simulink model "Simulink Circuit Design"  (R2024b)
settings: Solver=VariableStepAuto  StartTime=0.0  StopTime=1  RelTol=1e-3
libraries: spsSeriesRLCBranchLib x28, spsMosfetLib x24, spsVoltageMeasurementLib x10, spsCurrentMeasurementLib x7, spsDCVoltageSourceLib x4, spsGroundLib x1, sps_lib x1, spspowerguiLib x1
settings Model: Creator=davut.ertekin  LastModifiedBy=jraza
settings SolverCC: ZeroCrossAlgorithm=Adaptive
settings DebuggingCC: IgnoredZcDiagnostic=none
settings RTWCC: GPUComputeCapability=3.5

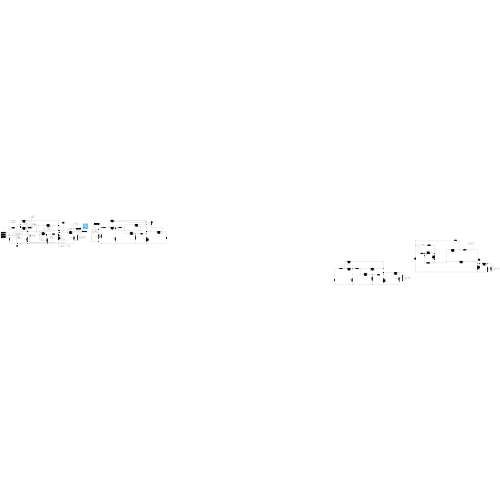
[thumbnail: Simulink's stored preview of the top-level diagram]
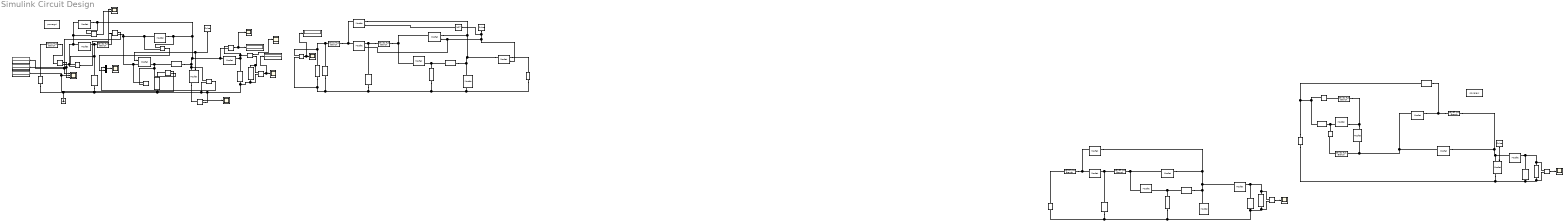
== system Simulink Circuit Design ==
  Co{3..4,8,14,16,19,21} (7 alike) : spsSeriesRLCBranchLib/Series RLC Branch  LConnTagsString=__new0  RConnTagsString=__new0  BranchType=C  Resistance=1  Inductance=1e-3  SetiL0=off  InitialCurrent=0  Capacitance=470e-6  Setx0=off  InitialVoltage=0  Measurements=None
  Co{2,5,9,15,20} (5 alike) : spsSeriesRLCBranchLib/Series RLC Branch  LConnTagsString=__new0  RConnTagsString=__new0  BranchType=C  Resistance=1  Inductance=1e-3  SetiL0=off  InitialCurrent=0  Capacitance=100e-6  Setx0=off  InitialVoltage=0  Measurements=None
  Current Measurement{,1..6} (7 alike) : spsCurrentMeasurementLib/Current Measurement  PhasorSimulation=off  OutputType=Complex  PSBequivalent=0
  DC Voltage Source : spsDCVoltageSourceLib/DC Voltage Source  Amplitude=300  Measurements=None
  DC Voltage Source2 : spsDCVoltageSourceLib/DC Voltage Source  Amplitude=24  Measurements=None
  DC Voltage Source4 : spsDCVoltageSourceLib/DC Voltage Source  Amplitude=24  Measurements=None
  DC Voltage Source6 : spsDCVoltageSourceLib/DC Voltage Source  Amplitude=24  Measurements=None
  Display{,1..5} (6 alike) : Display
  Ground : spsGroundLib/Ground  LConnTagsString=a
  L{1..3,7..9,14..15,17,19..21} (12 alike) : spsSeriesRLCBranchLib/Series RLC Branch  LConnTagsString=__new0  RConnTagsString=__new0  BranchType=L  Resistance=1  Inductance=330e-6  SetiL0=off  InitialCurrent=0  Capacitance=1e-6  Setx0=off  InitialVoltage=0  Measurements=None
  Load2 : spsSeriesRLCBranchLib/Series RLC Branch  LConnTagsString=__new0  RConnTagsString=__new0  BranchType=R  Resistance=200  Inductance=1e-3  SetiL0=off  InitialCurrent=0  Capacitance=1e-6  Setx0=off  InitialVoltage=0  Measurements=None
  Load3 : spsSeriesRLCBranchLib/Series RLC Branch  LConnTagsString=__new0  RConnTagsString=__new0  BranchType=R  Resistance=50  Inductance=1e-3  SetiL0=off  InitialCurrent=0  Capacitance=1e-6  Setx0=off  InitialVoltage=0  Measurements=None
  Load5 : spsSeriesRLCBranchLib/Series RLC Branch  LConnTagsString=__new0  RConnTagsString=__new0  BranchType=R  Resistance=300  Inductance=1e-3  SetiL0=off  InitialCurrent=0  Capacitance=1e-6  Setx0=off  InitialVoltage=0  Measurements=None
  Load7 : spsSeriesRLCBranchLib/Series RLC Branch  LConnTagsString=__new0  RConnTagsString=__new0  BranchType=R  Resistance=200  Inductance=1e-3  SetiL0=off  InitialCurrent=0  Capacitance=1e-6  Setx0=off  InitialVoltage=0  Measurements=None
  Mosfet{1..6,13..18,27..32,37..42} (24 alike) : spsMosfetLib/Mosfet  Ron=0.01  Lon=0  Rd=0.01  Vfd=0  IC=0  Rs=1e5  Cs=inf  Measurements=on
  Mux : Mux  Inputs=2
  NOT : Logic  Operator=NOT  IconShape=distinctive  AllPortsSameDT=off  OutDataTypeStr=boolean
  Pulse Generator1 : DiscretePulseGenerator  PulseType=Time based  Period=1/50000  PulseWidth=43
  Pulse Generator3 : DiscretePulseGenerator  PulseType=Time based  Period=1/50000  PulseWidth=80
  Pulse Generator4 : DiscretePulseGenerator  PulseType=Time based  Period=1/50000  PulseWidth=50.005
  Scope{,1,3..5,7..9} (8 alike) : Scope
  Scope2 : Scope  NumInputPorts=3
  Scope6 : Scope  NumInputPorts=2
  Vo{2..3,5,7} (4 alike) : spsVoltageMeasurementLib/Voltage Measurement  PhasorSimulation=off  OutputType=Complex  PSBequivalent=0
  Voltage Measurement{,1..5} (6 alike) : spsVoltageMeasurementLib/Voltage Measurement  PhasorSimulation=off  OutputType=Complex  PSBequivalent=0
  powergui : sps_lib/powergui  Priority=1  SimulationMode=Discrete  SampleTime=2e-6  frequency=60  Iterations=50  frequencyindice=0  Pbase=100e6  ErrMax=1e-4  UnitsV=kV  UnitsW=MW  buscounter=0  FunctionMessages=off  echomessages=off  EnableUseOfTLC=off  CurrentSourceSwitches=off  DisableSnubberDevices=off  DisableRonSwitches=off  DisableVfSwitches=off  DisplayEquations=off  AutomaticDiscreteSolvers=off  SolverType=Tustin/Backward Euler (TBE)  Interpol=off  ExternalGateDelay=off  methode=off  Ts=100  x0status=blocks  SPID=on  SwTol=0  HookPort=off  NonlinearTolerance=1e-4  nMaxIteration=100  ContinueOnMaxIteration=off  RestoreLinks=warning  ResistiveCurrentMeasurement=off  Frange=[0:2:500]  Ylog=off  Xlog=on  ShowGrid=off  save=off  variable=ZData  structure=0  ZoomFFT=off  StartTime=0.0  cycles=1  DisplayStyle=1  fundamental=60  FreqAxis=off  MaxFrequency=1000  frequencyindicesteady=1  RmsSteady=1  display=off
  powergui2 : spspowerguiLib/powergui  Priority=1  SimulationMode=Continuous  SampleTime=50e-6  frequency=60  Iterations=50  frequencyindice=0  Pbase=100e6  ErrMax=1e-4  UnitsV=kV  UnitsW=MW  buscounter=0  FunctionMessages=off  echomessages=off  EnableUseOfTLC=off  CurrentSourceSwitches=off  DisableSnubberDevices=off  DisableRonSwitches=off  DisableVfSwitches=off  DisplayEquations=off  AutomaticDiscreteSolvers=off  SolverType=Tustin/Backward Euler (TBE)  Interpol=off  ExternalGateDelay=off  methode=off  Ts=100  x0status=blocks  SPID=on  SwTol=0  HookPort=off  NonlinearTolerance=1e-4  nMaxIteration=100  ContinueOnMaxIteration=off  RestoreLinks=warning  ResistiveCurrentMeasurement=off  Frange=[0:2:500]  Ylog=off  Xlog=on  ShowGrid=off  save=off  variable=ZData  structure=0  ZoomFFT=off  StartTime=0.0  cycles=1  DisplayStyle=1  fundamental=60  FreqAxis=off  MaxFrequency=1000  frequencyindicesteady=1  RmsSteady=1  display=off
  wires:
  Pulse Generator3/1 -> Mosfet13/1
  Vo2/1 -> Scope1/1
  Vo5/1 -> Display4/1, Scope5/1
  Vo7/1 -> Scope7/1
  Pulse Generator4/1 -> Mosfet32/1, Mosfet29/1
  Voltage Measurement1/1 -> Mux/1
  Mux/1 -> Scope/1
  Voltage Measurement3/1 -> Mux/2
  Vo3/1 -> Display5/1, Scope4/1
  Pulse Generator1/1 -> Mosfet4/1, Mosfet1/1, Mosfet5/1, NOT/1
  NOT/1 -> Mosfet2/1
  Current Measurement/1 -> Display1/1, Scope2/3  "1"
  Current Measurement1/1 -> Display/1, Scope2/1  "2"
  Current Measurement2/1 -> Display2/1, Scope2/2  "3"
  Voltage Measurement5/1 -> Scope3/1, Display3/1
  Voltage Measurement2/1 -> Scope6/2  "1"
  Voltage Measurement/1 -> Scope6/1  "2"
  Current Measurement5/1 -> Scope8/1  "3"
  Current Measurement6/1 -> Scope9/1  "3"
  connections:
  L9/RConn1 -- Mosfet15/LConn1 -- Co9/LConn1
  Co5/RConn1 -- Current Measurement4/LConn1 -- Mosfet17/LConn1
  Mosfet18/LConn1 -- Mosfet15/RConn1 -- Mosfet16/RConn1 -- L8/RConn1
  Mosfet18/RConn1 -- L7/RConn1 -- Mosfet17/RConn1
  Vo2/LConn2 -- Mosfet13/RConn1 -- DC Voltage Source2/LConn1 -- Co8/RConn1 -- Load2/RConn1
  Mosfet14/RConn1 -- Mosfet13/LConn1 -- L9/LConn1 -- Mosfet16/LConn1
  DC Voltage Source2/RConn1 -- Co9/RConn1 -- Co5/LConn1 -- Current Measurement3/LConn1
  Mosfet14/LConn1 -- Co8/LConn1 -- Vo2/LConn1 -- Load2/LConn1
  L8/LConn1 -- Current Measurement4/RConn1
  L7/LConn1 -- Current Measurement3/RConn1
  Vo5/LConn2 -- Ground/LConn1 -- DC Voltage Source4/LConn1 -- Co16/RConn1 -- L17/LConn1 -- Voltage Measurement1/LConn2 -- Current Measurement5/RConn1 -- Co14/RConn1 -- Load5/RConn1
  Mosfet30/LConn1 -- Current Measurement6/LConn1 -- Voltage Measurement5/LConn1 -- Co14/LConn1
  Co15/LConn1 -- Current Measurement2/RConn1 -- Voltage Measurement4/LConn2 -- Mosfet32/RConn1
  Mosfet31/RConn1 -- Voltage Measurement4/LConn1 -- Mosfet32/LConn1 -- Current Measurement1/RConn1 -- Voltage Measurement3/LConn2
  Voltage Measurement1/LConn1 -- Voltage Measurement3/LConn1 -- Mosfet31/LConn1 -- Voltage Measurement2/LConn1 -- Mosfet28/LConn1 -- Voltage Measurement5/LConn2 -- Mosfet30/RConn1 -- Co15/RConn1 -- Mosfet29/LConn1
  Voltage Measurement/LConn2 -- Voltage Measurement2/LConn2 -- Mosfet28/RConn1 -- Mosfet27/RConn1 -- Current Measurement/RConn1
  Mosfet27/LConn1 -- Voltage Measurement/LConn1 -- Co16/LConn1 -- L15/LConn1
  DC Voltage Source4/RConn1 -- L14/LConn1
  L21/LConn1 -- Co21/RConn1 -- DC Voltage Source6/LConn1 -- Co19/RConn1 -- Load7/RConn1 -- Vo7/LConn2
  Mosfet41/LConn1 -- Mosfet38/LConn1 -- Mosfet40/RConn1 -- Co20/RConn1 -- Mosfet39/LConn1
  Co21/LConn1 -- L20/LConn1 -- Mosfet37/LConn1
  Mosfet40/LConn1 -- Co19/LConn1 -- Vo7/LConn1 -- Load7/LConn1
  L21/RConn1 -- Mosfet42/RConn1 -- Co20/LConn1
  L19/RConn1 -- Mosfet38/RConn1 -- Mosfet37/RConn1
  Mosfet41/RConn1 -- Mosfet42/LConn1 -- L20/RConn1
  DC Voltage Source6/RConn1 -- L19/LConn1
  L1/RConn1 -- Mosfet2/RConn1 -- Mosfet1/RConn1
  Mosfet4/LConn1 -- DC Voltage Source/RConn1
  Mosfet4/RConn1 -- Mosfet3/LConn1 -- Co2/RConn1 -- Mosfet2/LConn1 -- Mosfet5/LConn1
  Mosfet6/RConn1 -- L3/RConn1 -- Co2/LConn1
  L2/LConn1 -- Co3/LConn1 -- Mosfet1/LConn1
  Co3/RConn1 -- Vo3/LConn2 -- Load3/RConn1 -- Co4/RConn1 -- DC Voltage Source/LConn1 -- Mosfet3/RConn1 -- L3/LConn1
  Mosfet5/RConn1 -- Mosfet6/LConn1 -- L2/RConn1
  L1/LConn1 -- Vo3/LConn1 -- Load3/LConn1 -- Co4/LConn1
  L14/RConn1 -- Current Measurement/LConn1
  Current Measurement1/LConn1 -- L15/RConn1
  L17/RConn1 -- Current Measurement2/LConn1
  Load5/LConn1 -- Current Measurement6/RConn1 -- Vo5/LConn1
  Mosfet29/RConn1 -- Current Measurement5/LConn1
